simulink model "Tarea3Sim"  (R2022b)
settings: Solver=ode4  StartTime=0.0  StopTime=10.0  FixedStep=0.001  RelTol=1e-3
values from neighbouring files (symbols this model uses):
  b1 = 1000    [Tarea3Sim.m]
  f = 0    [Tarea3Sim.m]
  k1 = 16182    [Tarea3Sim.m]
  k2 = 19000    [Tarea3Sim.m]
  m1 = 290    [Tarea3Sim.m]
  m2 = 59    [Tarea3Sim.m]
  z1 = 0.05*sin(0.5*pi)    [Tarea3Sim.m]
settings Model: Creator=ferch  LastModifiedBy=ferch

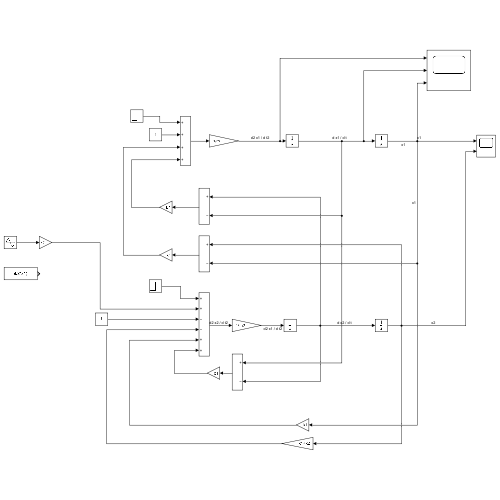
[thumbnail: Simulink's stored preview of the top-level diagram]
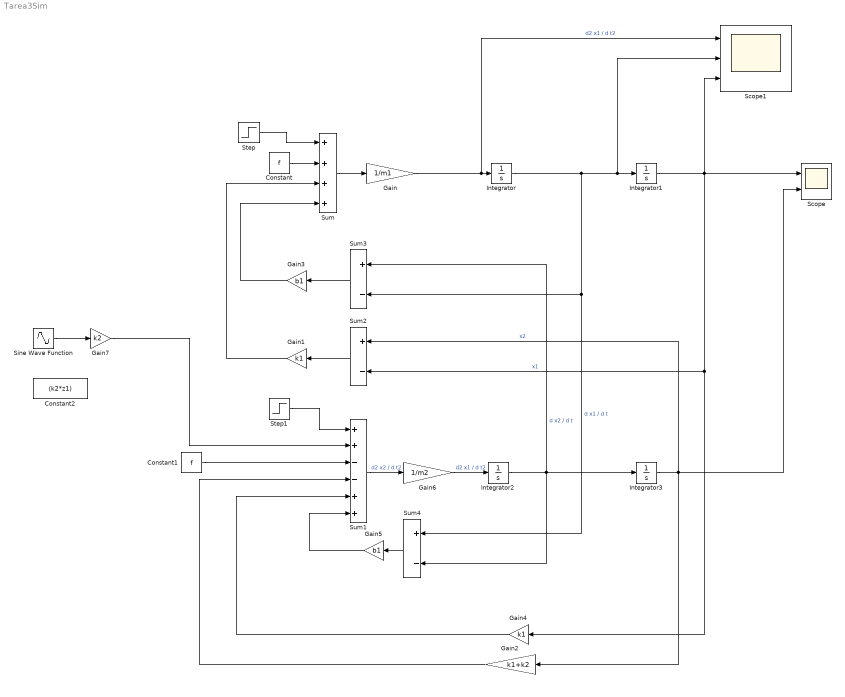
== system Tarea3Sim ==
  Constant : Constant  Value=f
  Constant1 : Constant  Value=f
  Constant2 : Constant  Value=(k2*z1)
  Gain : Gain  Gain=1/m1
  Gain1 : Gain  Gain=k1
  Gain2 : Gain  Gain=k1+k2
  Gain3 : Gain  Gain=b1
  Gain4 : Gain  Gain=k1
  Gain5 : Gain  Gain=b1
  Gain6 : Gain  Gain=1/m2
  Gain7 : Gain  Gain=k2
  Integrator{,1..3} (4 alike) : Integrator
  Scope : Scope  NumInputPorts=2
  Scope1 : Scope  NumInputPorts=3
  Sine Wave Function : Sin  Amplitude=0.05  Frequency=.5*pi  SampleTime=0
  Step : Step  SampleTime=0
  Step1 : Step  SampleTime=0
  Sum : Sum  Inputs=++++
  Sum1 : Sum  Inputs=++--++
  Sum2 : Sum  Inputs=+-
  Sum3 : Sum  Inputs=+-
  Sum4 : Sum  Inputs=+-
  wires:
  Sum/1 -> Gain/1
  Integrator/1 -> Sum4/1, Sum3/2, Integrator1/1, Scope1/2  "d x1 / d t"
  Integrator1/1 -> Sum2/2, Gain4/1, Scope/1, Scope1/3  "x1"
  Constant/1 -> Sum/2
  Sum1/1 -> Gain6/1  "d2 x2 / d t2"
  Integrator3/1 -> Gain2/1, Sum2/1, Scope/2  "x2"
  Integrator2/1 -> Sum3/1, Integrator3/1, Sum4/2  "d x2 / d t"
  Sum2/1 -> Gain1/1
  Gain1/1 -> Sum/3
  Sum3/1 -> Gain3/1
  Gain3/1 -> Sum/4
  Gain/1 -> Scope1/1, Integrator/1  "d2 x1 / d t2"
  Constant1/1 -> Sum1/3
  Gain2/1 -> Sum1/4
  Gain4/1 -> Sum1/5
  Sum4/1 -> Gain5/1
  Gain5/1 -> Sum1/6
  Gain6/1 -> Integrator2/1  "d2 x1 / d t2"
  Step/1 -> Sum/1
  Step1/1 -> Sum1/1
  Sine Wave Function/1 -> Gain7/1
  Gain7/1 -> Sum1/2
